simulink model "mwidefcncall"  (Simulink 6.3)
settings: Solver=FixedStepDiscrete  StartTime=0.0  StopTime=10.0  FixedStep=1  RelTol=1e-3
settings Model: CovMetricSettings=d  Creator=The MathWorks Inc.  LastModifiedBy=mshakeri  ExtModeEnableOpenProtocolUploading=on  ExtModeOpenProtocolUploadingEqualLengthVectors=off  ExtModeAutoUpdateStatusClock=off  StrictBusMsg=ErrorLevel1
settings DataIOCC: SignalLoggingName=logsOut
settings OptimizationCC: BlockReduction=off  BooleanDataType=off  InlineParams=on  InlineInvariantSignals=on
settings DebuggingCC: SignalResolutionControl=UseLocalSettings  SolverPrmCheckMsg=none
settings HardwareCC: TargetUnknown=on

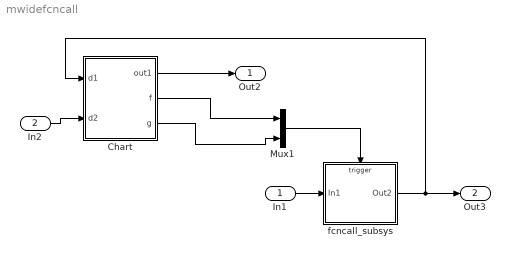
== system mwidefcncall ==
  In1 : Inport  Port=1  SampleTime=1
  In2 : Inport  Port=2  SampleTime=1
  Chart : Stateflow chart
  Mux1 : Mux  Inputs=2
  fcncall_subsys : Subsystem  TreatAsAtomicUnit=on
  Out2 : Outport
  Out3 : Outport  Port=2
  wires:
  Chart/3(g) -> Mux1/2
  fcncall_subsys/1(Out2) -> Out3/1, Chart/1(d1)
  Chart/1(out1) -> Out2/1
  In1/1 -> fcncall_subsys/1(In1)
  Chart/2(f) -> Mux1/1
  Mux1/1 -> fcncall_subsys/Trigger
  In2/1 -> Chart/2(d2)

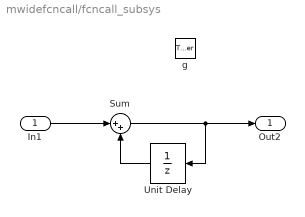
== system mwidefcncall/fcncall_subsys ==
  In1 : Inport  Port=1
  g : TriggerPort  TriggerType=function-call  StatesWhenEnabling=reset
  Sum : Sum  Inputs=|++  SaturateOnIntegerOverflow=on  InputSameDT=on
  Unit Delay : UnitDelay  Orientation=left  SampleTime=-1
  Out2 : Outport
  wires:
  In1/1 -> Sum/1
  Unit Delay/1 -> Sum/2
  Sum/1 -> Out2/1, Unit Delay/1

== stateflow chart Chart ==
  state one/
    entry: f; out1= d1+d2;
  state two/
    entry: g; out1=d1-d2;
  one -> two
  two -> one
  (default) -> one
  data: d1 input double; d2 input double; out1 output double
  events: f output FUNCTION_CALL_EVENT; g output FUNCTION_CALL_EVENT
